simulink model "halfCarModel"  (R2016b)
settings: Solver=FixedStepAuto  StartTime=0.0  StopTime=5  FixedStep=.005  RelTol=1e-3
settings Model: Creator=Devon  LastModifiedBy=Devon

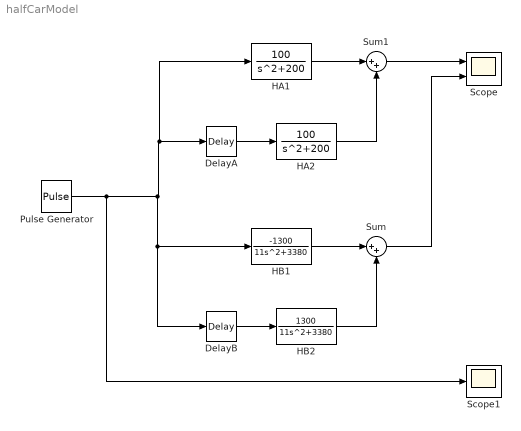
== system halfCarModel ==
  DelayA : TransportDelay  DelayTime=0.117117117117117
  DelayB : TransportDelay  DelayTime=0.117117117117117
  HA1 : TransferFcn  Numerator=100  Denominator=[1 0 200]
  HA2 : TransferFcn  Numerator=100  Denominator=[1 0 200]
  HB1 : TransferFcn  Numerator=-1300  Denominator=[11 0 3380]
  HB2 : TransferFcn  Numerator=1300  Denominator=[11 0 3380]
  Pulse Generator : DiscretePulseGenerator  PulseType=Time based  Period=10  PulseWidth=.001
  Scope : Scope  NumInputPorts=2
  Scope1 : Scope
  Sum : Sum  Inputs=|++
  Sum1 : Sum  Inputs=|++
  wires:
  Pulse Generator/1 -> Scope1/1, HB1/1, DelayB/1, HA1/1, DelayA/1
  Sum1/1 -> Scope/1
  Sum/1 -> Scope/2
  HA1/1 -> Sum1/1
  DelayA/1 -> HA2/1
  HA2/1 -> Sum1/2
  HB1/1 -> Sum/1
  HB2/1 -> Sum/2
  DelayB/1 -> HB2/1
